simulink model "Follower"  (R2024b)
settings: Solver=ode4  StartTime=0  StopTime=100  FixedStep=0.001  RelTol=1e-3
undefined symbols (not defined in the file or in its folder): DiscIntNeverNeededParam
libraries: simulink x22, vrlib x1
(part 3 of 4)

== matlab function Follower/Ardupilot Attitude Controller/Rate Controller/PID Yaw Rate/I/Integrator ==
  data: error input; integrator_out output; integrator input; limit_flg input; ki input; i_max input; dt input
function integrator_out = fcn(error, integrator, limit_flg, ki, i_max, dt)
% Code is based on AC_PID::update_i() in AC_PID.cpp.

% Check plausibility of input parameters
if (ki ~= 0 && dt > 0)
    % Only allow integration if limit is not set or the absolute sum of the
    % integrator would be reduced.
    if (~limit_flg || (integrator > 0 && error < 0) || (integrator < 0 && error > 0))
        integrator_out = integrator + error * ki * dt;
        integrator_out = max( min(integrator_out, i_max), -i_max);
    else % Otherwise, keep old integrator value
        integrator_out = integrator;
    end
else % Reset integrator if input parameters are not plausible
    integrator_out = 0.0;
end

== matlab function Follower/Ardupilot Attitude Controller/MATLAB Function ==
  data: euler input; q output
function q = fromEuler(euler)
% Computes quaternion from euler angle vector
% Based on QuaternionT<T>::from_euler()

q = zeros(4,1);
cr2 = cos(euler(1)*0.5);
cp2 = cos(euler(2)*0.5);
cy2 = cos(euler(3)*0.5);
sr2 = sin(euler(1)*0.5);
sp2 = sin(euler(2)*0.5);
sy2 = sin(euler(3)*0.5);

q(1) = cr2*cp2*cy2 + sr2*sp2*sy2;
q(2) = sr2*cp2*cy2 - cr2*sp2*sy2;
q(3) = cr2*sp2*cy2 + sr2*cp2*sy2;
q(4) = cr2*cp2*sy2 - sr2*sp2*cy2;

== matlab function Follower/Ardupilot Attitude Controller/Attitude Controller/input_euler_angle_roll_pitch_euler_rate_yaw()/Feedforward enabled/input shaping/input shaping pitch angle/MATLAB Function1 ==
  data: desiredAngVel input; targetAngVel input; eulerRateTar output; accelMax input; dt input; input_tc input
function eulerRateTar = input_shaping_ang_vel(desiredAngVel, targetAngVel, accelMax, dt, input_tc)
% Limits acceleration and deceleration of a velocity request
% Code based on AC_AttitudeControl::input_shaping_ang_vel()

if input_tc > 0
    % Calculate the acceleration to smoothly achieve rate. Jerk is not limited.
    errorRate = desiredAngVel - targetAngVel;
    desiredAngAccel = sqrt_controller(errorRate, 1.0/max(input_tc, 0.01), 0, dt);
    desiredAngVel = targetAngVel + desiredAngAccel * dt;
end

% Acceleration is limited directly to smooth the beginning of the curve
if accelMax > 0
    deltaAngVel = accelMax * dt;
    eulerRateTar = min(max(desiredAngVel, targetAngVel - deltaAngVel), targetAngVel + deltaAngVel);
else
    eulerRateTar = desiredAngVel;
end

== matlab function Follower/Ardupilot Attitude Controller/Attitude Controller/input_euler_angle_roll_pitch_euler_rate_yaw()/Feedforward enabled/input shaping/input shaping yaw rate/MATLAB Function1 ==
  data: desiredAngVel input; targetAngVel input; eulerRateTar output; accelMax input; dt input; input_tc input
function eulerRateTar = input_shaping_ang_vel(desiredAngVel, targetAngVel, accelMax, dt, input_tc)
% Limits acceleration and deceleration of a velocity request
% Code based on AC_AttitudeControl::input_shaping_ang_vel()

if input_tc > 0
    % Calculate the acceleration to smoothly achieve rate. Jerk is not limited.
    errorRate = desiredAngVel - targetAngVel;
    desiredAngAccel = sqrt_controller(errorRate, 1.0/max(input_tc, 0.01), 0, dt);
    desiredAngVel = targetAngVel + desiredAngAccel * dt;
end

% Acceleration is limited directly to smooth the beginning of the curve
if accelMax > 0
    deltaAngVel = accelMax * dt;
    eulerRateTar = min(max(desiredAngVel, targetAngVel - deltaAngVel), targetAngVel + deltaAngVel);
else
    eulerRateTar = desiredAngVel;
end

== matlab function Follower/Ardupilot Attitude Controller/Attitude Controller/input_euler_angle_roll_pitch_euler_rate_yaw()/MATLAB Function ==
  data: q input; roll output; pitch output; yaw output
function [roll, pitch, yaw] = toEuler(q)
% Function takes a quaternion and translates it into Euler angles
% Based on QuaternionT<T>::to_euler() and incorporates 
% QuaternionT<T>::get_euler_roll(), QuaternionT<T>::get_euler_pitch() and
% QuaternionT<T>::get_euler_yaw()

roll = atan2(2 * (q(1)*q(2) + q(3)*q(4)), 1 - 2*(q(2)*q(2) + q(3)*q(3)));
% Check if argument of asin is greater than 1 oder smaller than -1
% Based on safe_asin() in AP_MATH.cpp
xPitch = 2 * (q(1)*q(3) - q(4)*q(2));
if xPitch >= 1
    pitch = pi/2;
elseif xPitch <= -1
    pitch = -pi/2;
else
    pitch = asin(xPitch);
end
yaw = atan2(2*(q(1)*q(4) + q(2)*q(3)), 1 - 2*(q(3)*q(3) + q(4)*q(4)));

== matlab function Follower/Ardupilot Attitude Controller/Attitude Controller/input_euler_angle_roll_pitch_euler_rate_yaw()/Feedforward enabled/MATLAB Function ==
  data: eulerAngleTar input; eulerAccelMaxBF output; eulerAccelMaxEF input
function eulerAccelMaxBF = euler_accel_limit(eulerAngleTar, eulerAccelMaxEF)
% Translation of acceleration limits eulerAccelMax to the euler axis
% Code based on AC_AttitudeControl::euler_accel_limit()

sin_phi = max(min(abs(sin(eulerAngleTar(1))), 1), 0.1); % Sinus of roll angle
cos_phi = max(min(abs(cos(eulerAngleTar(1))), 1), 0.1);
sin_theta = max(min(abs(sin(eulerAngleTar(2))), 1), 0.1); % Sinus of pitch angle

eulerAccelMaxBF = zeros(3,1);
if eulerAccelMaxEF(1) == 0 || eulerAccelMaxEF(2) == 0 || eulerAccelMaxEF(3) == 0 || ...
   eulerAccelMaxEF(1) < 0 || eulerAccelMaxEF(2) < 0 || eulerAccelMaxEF(3) < 0 
    eulerAccelMaxBF(1) = eulerAccelMaxEF(1);
    eulerAccelMaxBF(2) = eulerAccelMaxEF(2);
    eulerAccelMaxBF(3) = eulerAccelMaxEF(3);
else
    eulerAccelMaxBF(1) = eulerAccelMaxEF(1);
    eulerAccelMaxBF(2) = min(eulerAccelMaxEF(2) / cos_phi, eulerAccelMaxEF(3) / sin_phi);
    eulerAccelMaxBF(3) = min(min(eulerAccelMaxEF(1) / sin_theta, eulerAccelMaxEF(2) / sin_phi), eulerAccelMaxEF(3) / cos_phi);
end

== matlab function Follower/Ardupilot Attitude Controller/Attitude Controller/input_euler_angle_roll_pitch_euler_rate_yaw()/Feedforward enabled/input shaping/input shaping roll angle/Square Root Controller ==
  data: err input; correction_rate output; p input; second_ord_lim input; dt input
function correction_rate = sqrt_controller(err, p, second_ord_lim, dt)
% The square root controller
% Code is taken from sqrt_controller(...) in AC_PosControl.cpp, line 296.

if (second_ord_lim < 0 || second_ord_lim == 0)
   correction_rate = err * p;
elseif (p == 0)
    % P term is zero, but second order limit is positive
    if (err > 0)
        correction_rate = sqrt(2.0 * second_ord_lim * err);
    elseif (err < 0)
        correction_rate = sqrt(2.0 * second_ord_lim * -err);
    else
        correction_rate = 0.0;
    end
else
    % P term and second order limit are positive, hence have been defined
    linear_dist = second_ord_lim / (p * p);
    % Check if error exceeds linear range of controller gain
    if (err > linear_dist)
        correction_rate = sqrt(2.0 * second_ord_lim * ( err - (linear_dist / 2.0) ));
    elseif (err < -linear_dist)
        correction_rate = -sqrt(2.0 * second_ord_lim * ( -err - (linear_dist / 2.0) ));
    else
        % Return linearly amplified correction if error is in linear range
        correction_rate = err * p;
    end
end

% Prevent oscillations by over-shooting the error correction in the last
% time step
if (dt ~= 0)
    correction_rate = max( min(correction_rate, abs(err) / dt), -abs(err) / dt);
end

== matlab function Follower/Ardupilot Attitude Controller/Attitude Controller/input_euler_angle_roll_pitch_euler_rate_yaw()/Feedforward enabled/input shaping/input shaping roll angle/MATLAB Function ==
  data: radIn input; radLim output
function radLim = wrapPi(radIn)
% Function to limit input angle in radian to [-pi pi].
% Code based on wrap_PI() and wrap_2PI() of AP_Math.cpp

% 1) Limit to [0 2pi]
radLim = mod(radIn, 2*pi);
if radLim < 0
    radLim = radLim + 2*pi;
end

% 2) Limit to [0 pi]
if radLim > pi
    radLim = radLim - 2*pi;
end

== matlab function Follower/Ardupilot Attitude Controller/Attitude Controller/input_euler_angle_roll_pitch_euler_rate_yaw()/Feedforward enabled/input shaping/input shaping roll angle/MATLAB Function1 ==
  data: desiredAngVel input; targetAngVel input; eulerRateTar output; accelMax input; dt input; input_tc input
function eulerRateTar = input_shaping_ang_vel(desiredAngVel, targetAngVel, accelMax, dt, input_tc)
% Limits acceleration and deceleration of a velocity request
% Code based on AC_AttitudeControl::input_shaping_ang_vel()

if input_tc > 0
    % Calculate the acceleration to smoothly achieve rate. Jerk is not limited.
    errorRate = desiredAngVel - targetAngVel;
    desiredAngAccel = sqrt_controller(errorRate, 1.0/max(input_tc, 0.01), 0, dt);
    desiredAngVel = targetAngVel + desiredAngAccel * dt;
end

% Acceleration is limited directly to smooth the beginning of the curve
if accelMax > 0
    deltaAngVel = accelMax * dt;
    eulerRateTar = min(max(desiredAngVel, targetAngVel - deltaAngVel), targetAngVel + deltaAngVel);
else
    eulerRateTar = desiredAngVel;
end

== matlab function Follower/Ardupilot Attitude Controller/Attitude Controller/input_euler_angle_roll_pitch_euler_rate_yaw()/Feedforward enabled/input shaping/input shaping pitch angle/MATLAB Function ==
  data: radIn input; radLim output
function radLim = wrapPi(radIn)
% Function to limit input angle in radian to [-pi pi].
% Code based on wrap_PI() and wrap_2PI() of AP_Math.cpp

% 1) Limit to [0 2pi]
radLim = mod(radIn, 2*pi);
if radLim < 0
    radLim = radLim + 2*pi;
end

% 2) Limit to [0 pi]
if radLim > pi
    radLim = radLim - 2*pi;
end

== matlab function Follower/Ardupilot Attitude Controller/Attitude Controller/input_euler_angle_roll_pitch_euler_rate_yaw()/reset yaw targets/MATLAB Function9 ==
  data: q1 input; qRes output; q2 input
function qRes = quatMult(q1, q2)
% Quaternion multiplication. Code based on QuaternionT<T>::operator*() in
% quaternion.cpp

qRes = zeros(4,1);
qRes(1) = q1(1)*q2(1) - q1(2)*q2(2) - q1(3)*q2(3) - q1(4)*q2(4);
qRes(2) = q1(1)*q2(2) + q1(2)*q2(1) + q1(3)*q2(4) - q1(4)*q2(3);
qRes(3) = q1(1)*q2(3) - q1(2)*q2(4) + q1(3)*q2(1) + q1(4)*q2(2);
qRes(4) = q1(1)*q2(4) + q1(2)*q2(3) - q1(3)*q2(2) + q1(4)*q2(1);

== matlab function Follower/Ardupilot Attitude Controller/Attitude Controller/input_euler_angle_roll_pitch_euler_rate_yaw()/Feedforward enabled/input shaping/input shaping pitch angle/Square Root Controller ==
  data: err input; correction_rate output; p input; second_ord_lim input; dt input
function correction_rate = sqrt_controller(err, p, second_ord_lim, dt)
% The square root controller
% Code is taken from sqrt_controller(...) in AC_PosControl.cpp, line 296.

if (second_ord_lim < 0 || second_ord_lim == 0)
   correction_rate = err * p;
elseif (p == 0)
    % P term is zero, but second order limit is positive
    if (err > 0)
        correction_rate = sqrt(2.0 * second_ord_lim * err);
    elseif (err < 0)
        correction_rate = sqrt(2.0 * second_ord_lim * -err);
    else
        correction_rate = 0.0;
    end
else
    % P term and second order limit are positive, hence have been defined
    linear_dist = second_ord_lim / (p * p);
    % Check if error exceeds linear range of controller gain
    if (err > linear_dist)
        correction_rate = sqrt(2.0 * second_ord_lim * ( err - (linear_dist / 2.0) ));
    elseif (err < -linear_dist)
        correction_rate = -sqrt(2.0 * second_ord_lim * ( -err - (linear_dist / 2.0) ));
    else
        % Return linearly amplified correction if error is in linear range
        correction_rate = err * p;
    end
end

% Prevent oscillations by over-shooting the error correction in the last
% time step
if (dt ~= 0)
    correction_rate = max( min(correction_rate, abs(err) / dt), -abs(err) / dt);
end

== matlab function Follower/Ardupilot Attitude Controller/Attitude Controller/input_euler_angle_roll_pitch_euler_rate_yaw()/Feedforward enabled/MATLAB Function1 ==
  data: eulerAngle input; angVelTar output; eulerRate input
function angVelTar = euler_rate_to_ang_vel(eulerAngle, eulerRate)
% This function converts euler angle derivatives (321 system) to an angular
% velocity vector. eulerAngle is the vector of the euler angles in rad and
% eulerRate is the vector of euler rates in rad/s
% Code based on AC_AttitudeControl::euler_rate_to_ang_vel()

sin_theta = sin(eulerAngle(2));
cos_theta = cos(eulerAngle(2));
sin_phi = sin(eulerAngle(1));
cos_phi = cos(eulerAngle(1));

angVelTar = zeros(3,1);
angVelTar(1) = eulerRate(1) - sin_theta * eulerRate(3);
angVelTar(2) = cos_phi * eulerRate(2) + sin_phi * cos_theta * eulerRate(3);
angVelTar(3) = -sin_phi * eulerRate(2) + cos_theta * cos_phi * eulerRate(3);

== matlab function Follower/Ardupilot Attitude Controller/Attitude Controller/input_euler_angle_roll_pitch_euler_rate_yaw()/reset yaw targets/MATLAB Function1 ==
  data: q input; roll output; pitch output; yaw output
function [roll, pitch, yaw] = toEuler(q)
% Function takes a quaternion and translates it into Euler angles
% Based on QuaternionT<T>::to_euler() and incorporates 
% QuaternionT<T>::get_euler_roll(), QuaternionT<T>::get_euler_pitch() and
% QuaternionT<T>::get_euler_yaw()

roll = atan2(2 * (q(1)*q(2) + q(3)*q(4)), 1 - 2*(q(2)*q(2) + q(3)*q(3)));
% Check if argument of asin is greater than 1 oder smaller than -1
% Based on safe_asin() in AP_MATH.cpp
xPitch = 2 * (q(1)*q(3) - q(4)*q(2));
if xPitch >= 1
    pitch = pi/2;
elseif xPitch <= -1
    pitch = -pi/2;
else
    pitch = asin(xPitch);
end
yaw = atan2(2*(q(1)*q(4) + q(2)*q(3)), 1 - 2*(q(3)*q(3) + q(4)*q(4)));

== matlab function Follower/Ardupilot Attitude Controller/Attitude Controller/input_euler_angle_roll_pitch_euler_rate_yaw()/Feedforward enabled/MATLAB Function2 ==
  data: angVelTar input; angVelTarLimited output; angVelRollMax input; angVelPitchMax input; angVelYawMax input
function angVelTarLimited = ang_vel_limit(angVelTar, angVelRollMax, angVelPitchMax, angVelYawMax)
% Limits angular velocity (rad/s) in body frame
% Code based on AC_AttitudeControl::ang_vel_limit()

angVelTarLimited = angVelTar;
if angVelRollMax == 0 || angVelPitchMax == 0
    if angVelRollMax ~= 0
        angVelTarLimited(1) = max(min(angVelTar(1), angVelRollMax), -angVelRollMax);
    end
    if angVelPitchMax ~= 0
        angVelTarLimited(2) = max(min(angVelTar(2), angVelPitchMax), -angVelPitchMax);
    end
else
    thrustVecAngVel = [angVelTar(1) / angVelRollMax; angVelTar(2) / angVelPitchMax];
    thrustVecLen = sqrt(thrustVecAngVel(1)^2 + thrustVecAngVel(2)^2);
    if thrustVecLen > 1
        angVelTarLimited(1) = thrustVecAngVel(1) * angVelRollMax / thrustVecLen;
        angVelTarLimited(2) = thrustVecAngVel(2) * angVelPitchMax / thrustVecLen;
    end
end
if angVelYawMax ~= 0
    angVelTarLimited(3) = max(min(angVelTar(3), angVelYawMax), -angVelYawMax);
end

== matlab function Follower/Ardupilot Attitude Controller/Attitude Controller/input_euler_angle_roll_pitch_euler_rate_yaw()/Feedforward enabled/MATLAB Function3 ==
  data: angVelBf input; eulerAngle input; eulerRate output
function eulerRate = ang_vel_to_euler_rate(angVelBf,eulerAngle)
% Function converts body-frame angular velocity into euler rate of desired
% attitude
% Based on AC_AttitudeControl::ang_vel_to_euler_rate()

sin_theta = sin(eulerAngle(2));
cos_theta = cos(eulerAngle(2));
sin_phi = sin(eulerAngle(1));
cos_phi = cos(eulerAngle(1));

eulerRate = zeros(3,1);
eulerRate(1) = angVelBf(1) + sin_phi * (sin_theta / cos_theta) * angVelBf(2) + cos_phi * (sin_theta / cos_theta) * angVelBf(3);
eulerRate(2) = cos_phi * angVelBf(2) - sin_phi * angVelBf(3);
eulerRate(3) = (sin_phi / cos_theta) * angVelBf(2) + (cos_phi / cos_theta) * angVelBf(3);

== matlab function Follower/Ardupilot Attitude Controller/Rate Controller/PID Pitch Rate/I/Integrator ==
  data: error input; integrator_out output; integrator input; limit_flg input; ki input; i_max input; dt input
function integrator_out = fcn(error, integrator, limit_flg, ki, i_max, dt)
% Code is based on AC_PID::update_i() in AC_PID.cpp.

% Check plausibility of input parameters
if (ki ~= 0 && dt > 0)
    % Only allow integration if limit is not set or the absolute sum of the
    % integrator would be reduced.
    if (~limit_flg || (integrator > 0 && error < 0) || (integrator < 0 && error > 0))
        integrator_out = integrator + error * ki * dt;
        integrator_out = max( min(integrator_out, i_max), -i_max);
    else % Otherwise, keep old integrator value
        integrator_out = integrator;
    end
else % Reset integrator if input parameters are not plausible
    integrator_out = 0.0;
end

== matlab function Follower/Ardupilot Attitude Controller/Attitude Controller/input_euler_angle_roll_pitch_euler_rate_yaw()/Feedforward disabled/MATLAB Function ==
  data: roll input; q output; pitch input; yaw input
function q = fromEuler(roll, pitch, yaw)
% Computes quaternion from euler angle vector
% Based on QuaternionT<T>::from_euler()

q = zeros(4,1);
cr2 = cos(roll*0.5);
cp2 = cos(pitch*0.5);
cy2 = cos(yaw*0.5);
sr2 = sin(roll*0.5);
sp2 = sin(pitch*0.5);
sy2 = sin(yaw*0.5);

q(1) = cr2*cp2*cy2 + sr2*sp2*sy2;
q(2) = sr2*cp2*cy2 - cr2*sp2*sy2;
q(3) = cr2*sp2*cy2 + sr2*cp2*sy2;
q(4) = cr2*cp2*sy2 - sr2*sp2*cy2;

== matlab function Follower/Ardupilot Attitude Controller/Attitude Controller/input_euler_angle_roll_pitch_euler_rate_yaw()/thrust_heading_rotation_angles()/thrust_vector_rotation_angles()/MATLAB Function ==
  data: q input; vecRot output; vec input
function vecRot = rotateByQuat(q, vec)
% Function rotates vector vec by quaternion q. Equivalent to converting the
% input quaternion to a rotation matrix and then multiplying it by the
% vector. This uses the formula
%
%    v2 = v1 + 2 q1 * qv x v1 + 2 qv x qv x v1
%
% where "x" is the cross product (explicitly inlined for performance below), 
% "q1" is the scalar part and "qv" is the vector part of this quaternion
% Code based on Vector3<T> QuaternionT<T>::operator*()

vecRot = vec;

% Compute and cache "qv x v1"
uv = [q(3) * vec(3) - q(4) * vec(2); q(4) * vec(1) - q(2) * vec(3); q(2) * vec(2) - q(3) * vec(1)];

uv(1) = uv(1) + uv(1);
uv(2) = uv(2) + uv(2);
uv(3) = uv(3) + uv(3);
vecRot(1) = vecRot(1) + q(1) * uv(1) + q(3) * uv(3) - q(4) * uv(2);
vecRot(2) = vecRot(2) + q(1) * uv(2) + q(4) * uv(1) - q(2) * uv(3);
vecRot(3) = vecRot(3) + q(1) * uv(3) + q(2) * uv(2) - q(3) * uv(1);

== matlab function Follower/Ardupilot Attitude Controller/Attitude Controller/input_euler_angle_roll_pitch_euler_rate_yaw()/thrust_heading_rotation_angles()/thrust_vector_rotation_angles()/MATLAB Function1 ==
  data: q input; vecRot output; vec input
function vecRot = rotateByQuat(q, vec)
% Function rotates vector vec by quaternion q. Equivalent to converting the
% input quaternion to a rotation matrix and then multiplying it by the
% vector. This uses the formula
%
%    v2 = v1 + 2 q1 * qv x v1 + 2 qv x qv x v1
%
% where "x" is the cross product (explicitly inlined for performance below), 
% "q1" is the scalar part and "qv" is the vector part of this quaternion
% Code based on Vector3<T> QuaternionT<T>::operator*()

vecRot = vec;

% Compute and cache "qv x v1"
uv = [q(3) * vec(3) - q(4) * vec(2); q(4) * vec(1) - q(2) * vec(3); q(2) * vec(2) - q(3) * vec(1)];

uv(1) = uv(1) + uv(1);
uv(2) = uv(2) + uv(2);
uv(3) = uv(3) + uv(3);
vecRot(1) = vecRot(1) + q(1) * uv(1) + q(3) * uv(3) - q(4) * uv(2);
vecRot(2) = vecRot(2) + q(1) * uv(2) + q(4) * uv(1) - q(2) * uv(3);
vecRot(3) = vecRot(3) + q(1) * uv(3) + q(2) * uv(2) - q(3) * uv(1);

== matlab function Follower/Ardupilot Attitude Controller/Attitude Controller/input_euler_angle_roll_pitch_euler_rate_yaw()/thrust_heading_rotation_angles()/thrust_vector_rotation_angles()/MATLAB Function2 ==
  data: thrustErrAngle input; rotVec input; rotVecNorm output
function rotVecNorm = normalizeVec(thrustErrAngle, rotVec)
% Function to normalize the thrust rotation vector. Divides the vector by
% its length or uses up-vector if thrust error angle is zero
rotVecNorm = zeros(3,1);
vecLen = sqrt(rotVec(1)^2 + rotVec(2)^2 + rotVec(3)^2);

if thrustErrAngle == 0 || vecLen == 0
    rotVecNorm = [0;0;-1];
else
    rotVecNorm(1) = rotVec(1) / vecLen;
    rotVecNorm(2) = rotVec(2) / vecLen;
    rotVecNorm(3) = rotVec(3) / vecLen;
end

== matlab function Follower/Ardupilot Attitude Controller/Attitude Controller/input_euler_angle_roll_pitch_euler_rate_yaw()/thrust_heading_rotation_angles()/thrust_vector_rotation_angles()/MATLAB Function3 ==
  data: q input; qInv output
function qInv = invertQuat(q)
% Function inverts the rotation of a quaternion.
% Code based on QuaternionT<T>::inverse(void)
% qInv = [q(1);-q(2);-q(3);-q(4)];
qInv = zeros(4,1);
qInv(1) = q(1);
qInv(2) = -q(2);
qInv(3) = -q(3);
qInv(4) = -q(4);

== matlab function Follower/Ardupilot Attitude Controller/Attitude Controller/input_euler_angle_roll_pitch_euler_rate_yaw()/thrust_heading_rotation_angles()/thrust_vector_rotation_angles()/MATLAB Function4 ==
  data: q input; vecRot output; vec input
function vecRot = rotateByQuat(q, vec)
% Function rotates vector vec by quaternion q. Equivalent to converting the
% input quaternion to a rotation matrix and then multiplying it by the
% vector. This uses the formula
%
%    v2 = v1 + 2 q1 * qv x v1 + 2 qv x qv x v1
%
% where "x" is the cross product (explicitly inlined for performance below), 
% "q1" is the scalar part and "qv" is the vector part of this quaternion
% Code based on Vector3<T> QuaternionT<T>::operator*()

vecRot = vec;

% Compute and cache "qv x v1"
uv = [q(3) * vec(3) - q(4) * vec(2); q(4) * vec(1) - q(2) * vec(3); q(2) * vec(2) - q(3) * vec(1)];

uv(1) = uv(1) + uv(1);
uv(2) = uv(2) + uv(2);
uv(3) = uv(3) + uv(3);
vecRot(1) = vecRot(1) + q(1) * uv(1) + q(3) * uv(3) - q(4) * uv(2);
vecRot(2) = vecRot(2) + q(1) * uv(2) + q(4) * uv(1) - q(2) * uv(3);
vecRot(3) = vecRot(3) + q(1) * uv(3) + q(2) * uv(2) - q(3) * uv(1);

== matlab function Follower/Ardupilot Attitude Controller/Attitude Controller/input_euler_angle_roll_pitch_euler_rate_yaw()/thrust_heading_rotation_angles()/thrust_vector_rotation_angles()/MATLAB Function5 ==
  data: axis input; angle input; q output
function q = fromAxisAngle(axis, angle)
% Create a quaternion from its axis-angle representation. The axis-vector
% must be of length 1 and the angle in radians.
% Based on QuaternionT<T>::from_axis_angle()

q = zeros(4,1);

if angle == 0
    q(1) = 1;
    q(2) = 0;
    q(3) = 0;
    q(4) = 0;
else
    st2 = sin(0.5*angle);
    q(1) = cos(0.5*angle);
    q(2) = axis(1) * st2;
    q(3) = axis(2) * st2;
    q(4) = axis(3) * st2;
end

== matlab function Follower/Ardupilot Attitude Controller/Attitude Controller/input_euler_angle_roll_pitch_euler_rate_yaw()/thrust_heading_rotation_angles()/thrust_vector_rotation_angles()/MATLAB Function6 ==
  data: q input; vec output
function vec = toAxisAngle(q)
% Converts the quaternion to a rotation vector. The direction represents
% the axis of rotation and the length represents the angle of rotation
% Code based on QuaternionT<T>::to_axis_angle()
l = sqrt(q(2)^2 + q(3)^2 + q(4)^2);

vec = [q(2);q(3);q(4)];

if l ~= 0
    vec = vec ./ l;
    mult = 2 * atan2(l, q(1));
    % The following lines are taken from wrap_pi() in AP_Math.cpp
    mult = mod(mult, 2*pi);
    if mult < 0
        mult = mult + 2*pi;
    end
    if mult > pi
        mult = mult - 2*pi;
    end

    vec = vec .* mult;
end

== matlab function Follower/Ardupilot Attitude Controller/Attitude Controller/input_euler_angle_roll_pitch_euler_rate_yaw()/thrust_heading_rotation_angles()/thrust_vector_rotation_angles()/MATLAB Function7 ==
  data: q input; qInv output
function qInv = invertQuat(q)
% Function inverts the rotation of a quaternion.
% Code based on QuaternionT<T>::inverse(void)
% qInv = [q(1);-q(2);-q(3);-q(4)];
qInv = zeros(4,1);
qInv(1) = q(1);
qInv(2) = -q(2);
qInv(3) = -q(3);
qInv(4) = -q(4);

== matlab function Follower/Ardupilot Attitude Controller/Attitude Controller/input_euler_angle_roll_pitch_euler_rate_yaw()/thrust_heading_rotation_angles()/thrust_vector_rotation_angles()/MATLAB Function8 ==
  data: q input; qInv output
function qInv = invertQuat(q)
% Function inverts the rotation of a quaternion.
% Code based on QuaternionT<T>::inverse(void)
qInv = [q(1);-q(2);-q(3);-q(4)];

== matlab function Follower/Ardupilot Attitude Controller/Attitude Controller/input_euler_angle_roll_pitch_euler_rate_yaw()/thrust_heading_rotation_angles()/thrust_vector_rotation_angles()/MATLAB Function9 ==
  data: q1 input; qRes output; q2 input
function qRes = quatMult(q1, q2)
% Quaternion multiplication. Code based on QuaternionT<T>::operator*() in
% quaternion.cpp

qRes = zeros(4,1);
qRes(1) = q1(1)*q2(1) - q1(2)*q2(2) - q1(3)*q2(3) - q1(4)*q2(4);
qRes(2) = q1(1)*q2(2) + q1(2)*q2(1) + q1(3)*q2(4) - q1(4)*q2(3);
qRes(3) = q1(1)*q2(3) - q1(2)*q2(4) + q1(3)*q2(1) + q1(4)*q2(2);
qRes(4) = q1(1)*q2(4) + q1(2)*q2(3) - q1(3)*q2(2) + q1(4)*q2(1);

== matlab function Follower/Ardupilot Attitude Controller/Attitude Controller/input_euler_angle_roll_pitch_euler_rate_yaw()/thrust_heading_rotation_angles()/thrust_vector_rotation_angles()/MATLAB Function10 ==
  data: q input; vec output
function vec = toAxisAngle(q)
% Converts the quaternion to a rotation vector. The direction represents
% the axis of rotation and the length represents the angle of rotation
% Code based on QuaternionT<T>::to_axis_angle()
l = sqrt(q(2)^2 + q(3)^2 + q(4)^2);

vec = [q(2);q(3);q(4)];

if l ~= 0
    vec = vec ./ l;
    mult = 2 * atan2(l, q(1));
    % The following lines are taken from wrap_pi() in AP_Math.cpp
    mult = mod(mult, 2*pi);
    if mult < 0
        mult = mult + 2*pi;
    end
    if mult > pi
        mult = mult - 2*pi;
    end

    vec = vec .* mult;
end

== matlab function Follower/Ardupilot Attitude Controller/Attitude Controller/input_euler_angle_roll_pitch_euler_rate_yaw()/thrust_heading_rotation_angles()/thrust_vector_rotation_angles()/MATLAB Function11 ==
  data: q1 input; qRes output; q2 input
function qRes = quatMult(q1, q2)
% Quaternion multiplication. Code based on QuaternionT<T>::operator*() in
% quaternion.cpp

qRes = zeros(4,1);
qRes(1) = q1(1)*q2(1) - q1(2)*q2(2) - q1(3)*q2(3) - q1(4)*q2(4);
qRes(2) = q1(1)*q2(2) + q1(2)*q2(1) + q1(3)*q2(4) - q1(4)*q2(3);
qRes(3) = q1(1)*q2(3) - q1(2)*q2(4) + q1(3)*q2(1) + q1(4)*q2(2);
qRes(4) = q1(1)*q2(4) + q1(2)*q2(3) - q1(3)*q2(2) + q1(4)*q2(1);

== matlab function Follower/Ardupilot Attitude Controller/Attitude Controller/input_euler_angle_roll_pitch_euler_rate_yaw()/thrust_heading_rotation_angles()/thrust_vector_rotation_angles()/MATLAB Function12 ==
  data: q1 input; qRes output; q2 input
function qRes = quatMult(q1, q2)
% Quaternion multiplication. Code based on QuaternionT<T>::operator*() in
% quaternion.cpp

qRes = zeros(4,1);
qRes(1) = q1(1)*q2(1) - q1(2)*q2(2) - q1(3)*q2(3) - q1(4)*q2(4);
qRes(2) = q1(1)*q2(2) + q1(2)*q2(1) + q1(3)*q2(4) - q1(4)*q2(3);
qRes(3) = q1(1)*q2(3) - q1(2)*q2(4) + q1(3)*q2(1) + q1(4)*q2(2);
qRes(4) = q1(1)*q2(4) + q1(2)*q2(3) - q1(3)*q2(2) + q1(4)*q2(1);

== matlab function Follower/Ardupilot Attitude Controller/Attitude Controller/input_euler_angle_roll_pitch_euler_rate_yaw()/thrust_heading_rotation_angles()/thrust_vector_rotation_angles()/MATLAB Function13 ==
  data: q input; qInv output
function qInv = invertQuat(q)
% Function inverts the rotation of a quaternion.
% Code based on QuaternionT<T>::inverse(void)
qInv = [q(1);-q(2);-q(3);-q(4)];

== matlab function Follower/Ardupilot Attitude Controller/Attitude Controller/input_euler_angle_roll_pitch_euler_rate_yaw()/thrust_heading_rotation_angles()/thrust_vector_rotation_angles()/MATLAB Function14 ==
  data: q input; qInv output
function qInv = invertQuat(q)
% Function inverts the rotation of a quaternion.
% Code based on QuaternionT<T>::inverse(void)
qInv = [q(1);-q(2);-q(3);-q(4)];

== matlab function Follower/MATLAB Function ==
  data: x input; U1 input; U2 input; U3 input; U4 input; xdot output; V input
function xdot = QuadrotorModel(x, U1, U2, U3, U4, V)
% x = (phi p theta q psi r x xdot y ydot z zdot)

%omega_bar = w1-w2+w3-w4
omega_bar = x(13) - x(14) + x(15) - x(16);
b = 280.19; beta0 = 189.63; beta1 = 6.0612; beta2 = 0.0122;

%initializing constants
m = 1.029; g = 9.81;
Ix = 15.48835e-3; Iy = Ix; Iz = 22.5656e-3;
Jr = 2.8385e-5;
% Jr = 0.0;
al = (Iy-Iz)/Ix; a3 = -Jr/Ix;
a4 = (Iz-Ix)/Iy; a6 = Jr/Iy;
a7 = (Ix-Iy)/Iz;
b1 = 1.1/Ix; b2 = 1.1/Iy; b3 = 0.2/Iz;
Ux = cos(x(1)) * sin(x(3)) * cos(x(5)) + sin(x(1)) * sin(x(5));
Uy = cos(x(1)) * sin(x(3)) * sin(x(5)) - sin(x(1)) * cos(x(5));
Uz = cos(x(1)) * cos(x(3));

% Introduce parameter uncertainty and distrubances
% Weak and Heavy Model:
% m = 1.2*m; U1 = 0.8*U1;
% Strong and Light Model:
% m = 0.8*m; U1 = 1.2*U1;

%Dynamics of the quadrotor
xdot = zeros(16,1);
xdot(1) = x(2) + x(4)*sin(x(1))*tan(x(3)) + x(6)*cos(x(1))*tan(x(3));
xdot(2) = al*x(4)*x(6) + a3*omega_bar*x(4) + b1*U2;
xdot(3) = x(4)*cos(x(1)) - x(6)*sin(x(1));
xdot(4) = a4*x(2)*x(6) + a6*omega_bar*x(2) + b2*U3;
xdot(5) = x(6)*(cos(x(1))/cos(x(3))) + x(4)*(sin(x(1))/cos(x(3)));
xdot(6) = a7*x(2)*x(4) + b3*U4;
xdot(7) = x(8);
xdot(8) = (Ux*U1)/m;
xdot(9) = x(10);
xdot(10) = (Uy*U1)/m;
xdot(11) = x(12);
xdot(12) = (Uz*U1)/m - g;

xdot(13) = b*V(1) - beta0 - beta1*x(13) - beta2*x(13)^2;
xdot(14) = b*V(2) - beta0 - beta1*x(14) - beta2*x(14)^2;
xdot(15) = b*V(3) - beta1 - beta1*x(15) - beta2*x(15)^2;
xdot(16) = b*V(4) - beta1 - beta1*x(16) - beta2*x(16)^2;

== matlab function Follower/Ardupilot Attitude Controller/Attitude Controller/input_euler_angle_roll_pitch_euler_rate_yaw()/thrust_heading_rotation_angles()/thrust_vector_rotation_angles()/MATLAB Function15 ==
  data: q1 input; qRes output; q2 input
function qRes = quatMult(q1, q2)
% Quaternion multiplication. Code based on QuaternionT<T>::operator*() in
% quaternion.cpp

qRes = zeros(4,1);
qRes(1) = q1(1)*q2(1) - q1(2)*q2(2) - q1(3)*q2(3) - q1(4)*q2(4);
qRes(2) = q1(1)*q2(2) + q1(2)*q2(1) + q1(3)*q2(4) - q1(4)*q2(3);
qRes(3) = q1(1)*q2(3) - q1(2)*q2(4) + q1(3)*q2(1) + q1(4)*q2(2);
qRes(4) = q1(1)*q2(4) + q1(2)*q2(3) - q1(3)*q2(2) + q1(4)*q2(1);

== matlab function Follower/Ardupilot Attitude Controller/Attitude Controller/input_euler_angle_roll_pitch_euler_rate_yaw()/thrust_heading_rotation_angles()/thrust_vector_rotation_angles()/MATLAB Function16 ==
  data: q input; vec output
function vec = toAxisAngle(q)
% Converts the quaternion to a rotation vector. The direction represents
% the axis of rotation and the length represents the angle of rotation
% Code based on QuaternionT<T>::to_axis_angle()
l = sqrt(q(2)^2 + q(3)^2 + q(4)^2);

vec = [q(2);q(3);q(4)];

if l ~= 0
    vec = vec ./ l;
    mult = 2 * atan2(l, q(1));
    % The following lines are taken from wrap_pi() in AP_Math.cpp
    mult = mod(mult, 2*pi);
    if mult < 0
        mult = mult + 2*pi;
    end
    if mult > pi
        mult = mult - 2*pi;
    end

    vec = vec .* mult;
end

== matlab function Follower/Ardupilot Attitude Controller/Attitude Controller/input_euler_angle_roll_pitch_euler_rate_yaw()/thrust_heading_rotation_angles()/Yaw error limitation/Yaw limiting and recalculation of attitudeTarget/MATLAB Function ==
  data: radIn input; radLim output
function radLim = wrapPi(radIn)
% Function to limit input angle in radian to [-pi pi].
% Code based on wrap_PI() and wrap_2PI() of AP_Math.cpp

% 1) Limit to [0 2pi]
radLim = mod(radIn, 2*pi);
if radLim < 0
    radLim = radLim + 2*pi;
end

% 2) Limit to [0 pi]
if radLim > pi
    radLim = radLim - 2*pi;
end

== matlab function Follower/Ardupilot Attitude Controller/Attitude Controller/input_euler_angle_roll_pitch_euler_rate_yaw()/thrust_heading_rotation_angles()/Yaw error limitation/Yaw limiting and recalculation of attitudeTarget/MATLAB Function5 ==
  data: vec input; q output
function q = fromAxisAngle(vec)
% Create a quaternion from its axis-angle representation. Just the rotation
% vector is given as input.
% Based on QuaternionT<T>::from_axis_angle(Vector3<T>)

q = zeros(4,1);
angle = sqrt(vec(1)^2 + vec(2)^2 + vec(3)^2);

if angle == 0
    q(1) = 1;
    q(2) = 0;
    q(3) = 0;
    q(4) = 0;
else
    axis = vec ./ angle;
    % The following lines are based on QuaternionT<T>::from_axis_angle(const Vector3<T> &axis, T theta)
    if angle == 0
        q(1) = 1;
        q(2) = 0;
        q(3) = 0;
        q(4) = 0;
    else
        st2 = sin(0.5*angle);
        q(1) = cos(0.5*angle);
        q(2) = axis(1) * st2;
        q(3) = axis(2) * st2;
        q(4) = axis(3) * st2;
    end
end

== matlab function Follower/Ardupilot Attitude Controller/Attitude Controller/input_euler_angle_roll_pitch_euler_rate_yaw()/thrust_heading_rotation_angles()/Yaw error limitation/Yaw limiting and recalculation of attitudeTarget/MATLAB Function9 ==
  data: q1 input; qRes output; q2 input
function qRes = quatMult(q1, q2)
% Quaternion multiplication. Code based on QuaternionT<T>::operator*() in
% quaternion.cpp

qRes = zeros(4,1);
qRes(1) = q1(1)*q2(1) - q1(2)*q2(2) - q1(3)*q2(3) - q1(4)*q2(4);
qRes(2) = q1(1)*q2(2) + q1(2)*q2(1) + q1(3)*q2(4) - q1(4)*q2(3);
qRes(3) = q1(1)*q2(3) - q1(2)*q2(4) + q1(3)*q2(1) + q1(4)*q2(2);
qRes(4) = q1(1)*q2(4) + q1(2)*q2(3) - q1(3)*q2(2) + q1(4)*q2(1);

== matlab function Follower/Ardupilot Attitude Controller/Attitude Controller/input_euler_angle_roll_pitch_euler_rate_yaw()/thrust_heading_rotation_angles()/Yaw error limitation/Yaw limiting and recalculation of attitudeTarget/MATLAB Function1 ==
  data: q1 input; qRes output; q2 input
function qRes = quatMult(q1, q2)
% Quaternion multiplication. Code based on QuaternionT<T>::operator*() in
% quaternion.cpp

qRes = zeros(4,1);
qRes(1) = q1(1)*q2(1) - q1(2)*q2(2) - q1(3)*q2(3) - q1(4)*q2(4);
qRes(2) = q1(1)*q2(2) + q1(2)*q2(1) + q1(3)*q2(4) - q1(4)*q2(3);
qRes(3) = q1(1)*q2(3) - q1(2)*q2(4) + q1(3)*q2(1) + q1(4)*q2(2);
qRes(4) = q1(1)*q2(4) + q1(2)*q2(3) - q1(3)*q2(2) + q1(4)*q2(1);

== matlab function Follower/Ardupilot Attitude Controller/Attitude Controller/input_euler_angle_roll_pitch_euler_rate_yaw()/update_ang_vel_target_from_att_error()/Calc angular velocity target roll/Square Root Controller ==
  data: err input; correction_rate output; p input; second_ord_lim input; dt input
function correction_rate = sqrt_controller(err, p, second_ord_lim, dt)
% The square root controller
% Code is taken from sqrt_controller(...) in AC_PosControl.cpp, line 296.

if (second_ord_lim < 0 || second_ord_lim == 0)
   correction_rate = err * p;
elseif (p == 0)
    % P term is zero, but second order limit is positive
    if (err > 0)
        correction_rate = sqrt(2.0 * second_ord_lim * err);
    elseif (err < 0)
        correction_rate = sqrt(2.0 * second_ord_lim * -err);
    else
        correction_rate = 0.0;
    end
else
    % P term and second order limit are positive, hence have been defined
    linear_dist = second_ord_lim / (p * p);
    % Check if error exceeds linear range of controller gain
    if (err > linear_dist)
        correction_rate = sqrt(2.0 * second_ord_lim * ( err - (linear_dist / 2.0) ));
    elseif (err < -linear_dist)
        correction_rate = -sqrt(2.0 * second_ord_lim * ( -err - (linear_dist / 2.0) ));
    else
        % Return linearly amplified correction if error is in linear range
        correction_rate = err * p;
    end
end

% Prevent oscillations by over-shooting the error correction in the last
% time step
if (dt ~= 0)
    correction_rate = max( min(correction_rate, abs(err) / dt), -abs(err) / dt);
end

== matlab function Follower/Ardupilot Attitude Controller/Attitude Controller/input_euler_angle_roll_pitch_euler_rate_yaw()/update_ang_vel_target_from_att_error()/Calc angular velocity target pitch/Square Root Controller ==
  data: err input; correction_rate output; p input; second_ord_lim input; dt input
function correction_rate = sqrt_controller(err, p, second_ord_lim, dt)
% The square root controller
% Code is taken from sqrt_controller(...) in AC_PosControl.cpp, line 296.

if (second_ord_lim < 0 || second_ord_lim == 0)
   correction_rate = err * p;
elseif (p == 0)
    % P term is zero, but second order limit is positive
    if (err > 0)
        correction_rate = sqrt(2.0 * second_ord_lim * err);
    elseif (err < 0)
        correction_rate = sqrt(2.0 * second_ord_lim * -err);
    else
        correction_rate = 0.0;
    end
else
    % P term and second order limit are positive, hence have been defined
    linear_dist = second_ord_lim / (p * p);
    % Check if error exceeds linear range of controller gain
    if (err > linear_dist)
        correction_rate = sqrt(2.0 * second_ord_lim * ( err - (linear_dist / 2.0) ));
    elseif (err < -linear_dist)
        correction_rate = -sqrt(2.0 * second_ord_lim * ( -err - (linear_dist / 2.0) ));
    else
        % Return linearly amplified correction if error is in linear range
        correction_rate = err * p;
    end
end

% Prevent oscillations by over-shooting the error correction in the last
% time step
if (dt ~= 0)
    correction_rate = max( min(correction_rate, abs(err) / dt), -abs(err) / dt);
end

== matlab function Follower/Ardupilot Attitude Controller/Attitude Controller/input_euler_angle_roll_pitch_euler_rate_yaw()/update_ang_vel_target_from_att_error()/Calc angular velocity target yaw/Square Root Controller ==
  data: err input; correction_rate output; p input; second_ord_lim input; dt input
function correction_rate = sqrt_controller(err, p, second_ord_lim, dt)
% The square root controller
% Code is taken from sqrt_controller(...) in AC_PosControl.cpp, line 296.

if (second_ord_lim < 0 || second_ord_lim == 0)
   correction_rate = err * p;
elseif (p == 0)
    % P term is zero, but second order limit is positive
    if (err > 0)
        correction_rate = sqrt(2.0 * second_ord_lim * err);
    elseif (err < 0)
        correction_rate = sqrt(2.0 * second_ord_lim * -err);
    else
        correction_rate = 0.0;
    end
else
    % P term and second order limit are positive, hence have been defined
    linear_dist = second_ord_lim / (p * p);
    % Check if error exceeds linear range of controller gain
    if (err > linear_dist)
        correction_rate = sqrt(2.0 * second_ord_lim * ( err - (linear_dist / 2.0) ));
    elseif (err < -linear_dist)
        correction_rate = -sqrt(2.0 * second_ord_lim * ( -err - (linear_dist / 2.0) ));
    else
        % Return linearly amplified correction if error is in linear range
        correction_rate = err * p;
    end
end

% Prevent oscillations by over-shooting the error correction in the last
% time step
if (dt ~= 0)
    correction_rate = max( min(correction_rate, abs(err) / dt), -abs(err) / dt);
end

== matlab function Follower/Ardupilot Attitude Controller/Attitude Controller/input_euler_angle_roll_pitch_euler_rate_yaw()/MATLAB Function2 ==
  data: angVel input; angVelLimited output; angVelRollMax input; angVelPitchMax input; angVelYawMax input
function angVelLimited = ang_vel_limit(angVel, angVelRollMax, angVelPitchMax, angVelYawMax)
% Limits angular velocity (rad/s) in body frame
% Code based on AC_AttitudeControl::ang_vel_limit()

angVelLimited = angVel;
if angVelRollMax == 0 || angVelPitchMax == 0
    if angVelRollMax ~= 0
        angVelLimited(1) = max(min(angVel(1), angVelRollMax), -angVelRollMax);
    end
    if angVelPitchMax ~= 0
        angVelLimited(2) = max(min(angVel(2), angVelPitchMax), -angVelPitchMax);
    end
else
    thrustVecAngVel = [angVel(1) / angVelRollMax; angVel(2) / angVelPitchMax];
    thrustVecLen = sqrt(thrustVecAngVel(1)^2 + thrustVecAngVel(2)^2);
    if thrustVecLen > 1
        angVelLimited(1) = thrustVecAngVel(1) * angVelRollMax / thrustVecLen;
        angVelLimited(2) = thrustVecAngVel(2) * angVelPitchMax / thrustVecLen;
    end
end
if angVelYawMax ~= 0
    angVelLimited(3) = max(min(angVel(3), angVelYawMax), -angVelYawMax);
end

== matlab function Follower/Ardupilot Attitude Controller/Attitude Controller/input_euler_angle_roll_pitch_euler_rate_yaw()/MATLAB Function7 ==
  data: q input; qInv output
function qInv = invertQuat(q)
% Function inverts the rotation of a quaternion.
% Code based on QuaternionT<T>::inverse(void)
% qInv = [q(1);-q(2);-q(3);-q(4)];
qInv = zeros(4,1);
qInv(1) = q(1);
qInv(2) = -q(2);
qInv(3) = -q(3);
qInv(4) = -q(4);

== matlab function Follower/Ardupilot Attitude Controller/Attitude Controller/input_euler_angle_roll_pitch_euler_rate_yaw()/MATLAB Function11 ==
  data: q1 input; qRes output; q2 input
function qRes = quatMult(q1, q2)
% Quaternion multiplication. Code based on QuaternionT<T>::operator*() in
% quaternion.cpp

qRes = zeros(4,1);
qRes(1) = q1(1)*q2(1) - q1(2)*q2(2) - q1(3)*q2(3) - q1(4)*q2(4);
qRes(2) = q1(1)*q2(2) + q1(2)*q2(1) + q1(3)*q2(4) - q1(4)*q2(3);
qRes(3) = q1(1)*q2(3) - q1(2)*q2(4) + q1(3)*q2(1) + q1(4)*q2(2);
qRes(4) = q1(1)*q2(4) + q1(2)*q2(3) - q1(3)*q2(2) + q1(4)*q2(1);

== matlab function Follower/Ardupilot Attitude Controller/Attitude Controller/input_euler_angle_roll_pitch_euler_rate_yaw()/MATLAB Function4 ==
  data: q input; vecRot output; vec input
function vecRot = rotateByQuat(q, vec)
% Function rotates vector vec by quaternion q. Equivalent to converting the
% input quaternion to a rotation matrix and then multiplying it by the
% vector. This uses the formula
%
%    v2 = v1 + 2 q1 * qv x v1 + 2 qv x qv x v1
%
% where "x" is the cross product (explicitly inlined for performance below), 
% "q1" is the scalar part and "qv" is the vector part of this quaternion
% Code based on Vector3<T> QuaternionT<T>::operator*()

vecRot = vec;

% Compute and cache "qv x v1"
uv = [q(3) * vec(3) - q(4) * vec(2); q(4) * vec(1) - q(2) * vec(3); q(2) * vec(2) - q(3) * vec(1)];

uv(1) = uv(1) + uv(1);
uv(2) = uv(2) + uv(2);
uv(3) = uv(3) + uv(3);
vecRot(1) = vecRot(1) + q(1) * uv(1) + q(3) * uv(3) - q(4) * uv(2);
vecRot(2) = vecRot(2) + q(1) * uv(2) + q(4) * uv(1) - q(2) * uv(3);
vecRot(3) = vecRot(3) + q(1) * uv(3) + q(2) * uv(2) - q(3) * uv(1);

== matlab function Follower/Ardupilot Attitude Controller/Attitude Controller/input_euler_angle_roll_pitch_euler_rate_yaw()/Add feedforward to angVelBody/MATLAB Function ==
  data: angVelBodyFeedforward input; angVelBodyNew output; angVelBodyIn input; thrustErrorAngle input; yawRateAct input; maxThrustErrorAngle4YawCorr input; feedforwardScaler output
function [angVelBodyNew, feedforwardScaler] = addFeedforwardToTargetAngVel(angVelBodyFeedforward, angVelBodyIn, thrustErrorAngle, yawRateAct, maxThrustErrorAngle4YawCorr)
% Function smoothly adds feedforward angular velocity and yaw input to
% target angular velocity.
% Code based on AC_AttitudeControl::attitude_controller_run_quat()

angVelBodyNew = angVelBodyIn;

feedforwardScaler = 1;
if thrustErrorAngle > 2 * maxThrustErrorAngle4YawCorr
    % thrustErrorAngle too large. Set target yaw rate to actual rate. Do not
    % add feedforward.
    angVelBodyNew(3) = yawRateAct;
elseif thrustErrorAngle > maxThrustErrorAngle4YawCorr
    % thrustErrorAngle still large. Add feedforward values smoothly.
    feedforwardScaler = 1 - (thrustErrorAngle - maxThrustErrorAngle4YawCorr) / maxThrustErrorAngle4YawCorr;
    angVelBodyNew(1) = angVelBodyNew(1) + angVelBodyFeedforward(1) * feedforwardScaler;
    angVelBodyNew(2) = angVelBodyNew(2) + angVelBodyFeedforward(2) * feedforwardScaler;
    angVelBodyNew(3) = angVelBodyNew(3) + angVelBodyFeedforward(3);
    angVelBodyNew(3) = yawRateAct * (1 - feedforwardScaler) + angVelBodyNew(3) * feedforwardScaler;
else
    % thrustErrorAngle small enough to add feedforward values to target
    % angular rates of controller without smoothing.
    angVelBodyNew = angVelBodyNew + angVelBodyFeedforward;
end

== matlab function Follower/High-gain Observer/MATLAB Function2 ==
  data: x input; zintg input; xhatdot output; xhat input; U1 input; UxUyact output
function [xhatdot, UxUyact] = HighGainObserver(x, zintg, xhat, U1)

% Set the main design parameters of the High Gain Observer
% Note 1: The value of epsilon is a balance between rejecting modeling errors
% and disturbances (small) and sensitivity to measurement noise (large)
% Note 2: The choice of alpha is less important as long as the roots of 
% s^2 + alpha1 * s + alpha2 = 0 are in the open left-half plane
epsilon_x = 0.025;
alpha_x1 = 1.0;
alpha_x2 = 0.5;

epsilon_y = 0.025;
alpha_y1 = 1.0;
alpha_y2 = 0.5;

epsilon_z = 0.025;
alpha_z1 = 2.0;
alpha_z2 = 0.5;

% Calculate the h1 and h2 of the observer for x, y and z
h1_x = alpha_x1 / epsilon_x;
h2_x = alpha_x2 / (epsilon_x^2);
h1_y = alpha_y1 / epsilon_y;
h2_y = alpha_y2 / (epsilon_y^2);
h1_z = alpha_z1 / epsilon_z;
h22_z = alpha_z2 / (epsilon_z^2);
h21_z = 2 * h22_z;

% Calculate the values of Ux, Uy and Uz based on phi, theta and psi
% Note: x = (phi phidot theta thetadot psi psidot x xdot y ydot z zdot)
Ux = cos(x(1)) * sin(x(3)) * cos(x(5)) + sin(x(1)) * sin(x(5));
Uy = cos(x(1)) * sin(x(3)) * sin(x(5)) - sin(x(1)) * cos(x(5));
Uz = cos(x(1)) * cos(x(3));
UxUyact = [Ux Uy];

% Update xhatdot based on the observer model
% xhat = (x xdot y ydot z zdot)
g = 9.81; m0 = 1.029; % Nominal mass
xhatdot = zeros(6, 1); 

xhatdot(1) = xhat(2) + h1_x * (x(7) - xhat(1));
xhatdot(2) = U1 * Ux / m0 + h2_x * (x(7) - xhat(1));
xhatdot(3) = xhat(4) + h1_y * (x(9) - xhat(3));
xhatdot(4) = U1 * Uy / m0 + h2_y * (x(9) - xhat(3));
xhatdot(5) = xhat(6) + h1_z * (x(11) - xhat(5));
xhatdot(6) = U1 * Uz / m0 - g + + h21_z * zintg + h22_z * (x(11) - xhat(5));

== matlab function Follower/Ardupilot Attitude Controller/Attitude Controller/input_euler_angle_roll_pitch_euler_rate_yaw()/Update attitudeTarget/MATLAB Function ==
  data: q input; qNorm output
function qNorm = normalizeQuat(q)
% Function to normalze a quaternion. Code based on
% QuaternionT<T>::normalize()

quatLen = sqrt(q(1)^2 + q(2)^2 + q(3)^2 + q(4)^2);
if quatLen ~= 0
    qNorm = q ./ quatLen;
else
    qNorm = q;
end

== matlab function Follower/Ardupilot Attitude Controller/Attitude Controller/input_euler_angle_roll_pitch_euler_rate_yaw()/Update attitudeTarget/Rotate target attitude/MATLAB Function5 ==
  data: vec input; q output
function q = fromAxisAngle(vec)
% Create a quaternion from its axis-angle representation. Just the rotation
% vector is given as input.
% Based on QuaternionT<T>::from_axis_angle(Vector3<T>)

q = zeros(4,1);
angle = sqrt(vec(1)^2 + vec(2)^2 + vec(3)^2);

if angle == 0
    q(1) = 1;
    q(2) = 0;
    q(3) = 0;
    q(4) = 0;
else
    axis = vec ./ angle;
    % The following lines are based on QuaternionT<T>::from_axis_angle(const Vector3<T> &axis, T theta)
    if angle == 0
        q(1) = 1;
        q(2) = 0;
        q(3) = 0;
        q(4) = 0;
    else
        st2 = sin(0.5*angle);
        q(1) = cos(0.5*angle);
        q(2) = axis(1) * st2;
        q(3) = axis(2) * st2;
        q(4) = axis(3) * st2;
    end
end

== matlab function Follower/Ardupilot Attitude Controller/Attitude Controller/input_euler_angle_roll_pitch_euler_rate_yaw()/Update attitudeTarget/Rotate target attitude/MATLAB Function1 ==
  data: q1 input; qRes output; q2 input
function qRes = quatMult(q1, q2)
% Quaternion multiplication. Code based on QuaternionT<T>::operator*() in
% quaternion.cpp

qRes = zeros(4,1);
qRes(1) = q1(1)*q2(1) - q1(2)*q2(2) - q1(3)*q2(3) - q1(4)*q2(4);
qRes(2) = q1(1)*q2(2) + q1(2)*q2(1) + q1(3)*q2(4) - q1(4)*q2(3);
qRes(3) = q1(1)*q2(3) - q1(2)*q2(4) + q1(3)*q2(1) + q1(4)*q2(2);
qRes(4) = q1(1)*q2(4) + q1(2)*q2(3) - q1(3)*q2(2) + q1(4)*q2(1);

== matlab function Follower/Ardupilot Attitude Controller/Attitude Controller/input_euler_angle_roll_pitch_euler_rate_yaw()/reset yaw targets/MATLAB Function5 ==
  data: vec input; q output
function q = fromAxisAngle(vec)
% Create a quaternion from its axis-angle representation. Just the rotation
% vector is given as input.
% Based on QuaternionT<T>::from_axis_angle(Vector3<T>)

q = zeros(4,1);
angle = single(sqrt(vec(1)^2 + vec(2)^2 + vec(3)^2));

if angle == 0
    q(1) = single(1);
    q(2) = single(0);
    q(3) = single(0);
    q(4) = single(0);
else
    axis = vec ./ angle;
    % The following lines are based on QuaternionT<T>::from_axis_angle(const Vector3<T> &axis, T theta)
    if angle == 0
        q(1) = single(1);
        q(2) = single(0);
        q(3) = single(0);
        q(4) = single(0);
    else
        st2 = single(sin(0.5*angle));
        q(1) = single(cos(0.5*angle));
        q(2) = axis(1) * st2;
        q(3) = axis(2) * st2;
        q(4) = axis(3) * st2;
    end
end
